simulink model "PolarCinematica2015"  (R2015a)
settings: Solver=ode45  SolverMode=SingleTasking  StartTime=0.0  StopTime=Tfinal  RelTol=1e-3
values from neighbouring files (symbols this model uses):
  Tem = 0.001    [circular.m]
undefined symbols (not defined in the file or in its folder): Diferencia, mgd_Polar, mgi_Polar
libraries: simulink x1
settings Model: CovMetricSettings=dwe  CovHtmlReporting=off  covSaveCumulativeToWorkspaceVar=off  CovSaveSingleToWorkspaceVar=off  CovExternalEMLEnable=on  Creator=Shadow  LastModifiedBy=Shadow
settings DataIOCC: LimitDataPoints=off  SaveFormat=Dataset  ReturnWorkspaceOutputs=on
settings DebuggingCC: SFUnexpectedBacktrackingDiag=error  SFNoUnconditionalDefaultTransitionDiag=error
settings HardwareCC: ProdBitPerPointer=64  ProdLargestAtomicFloat=Float  ProdIntDivRoundTo=Zero  ProdEndianess=LittleEndian  ProdHWDeviceType=Specified
settings ModelReferenceCC: PropagateSignalLabelsOutOfModel=on
settings SFSimCC: SimUseLocalCustomCode=on
settings RTWCC: RTWUseLocalCustomCode=on
settings GRTTargetCC: TargetLangStandard=C99 (ISO)

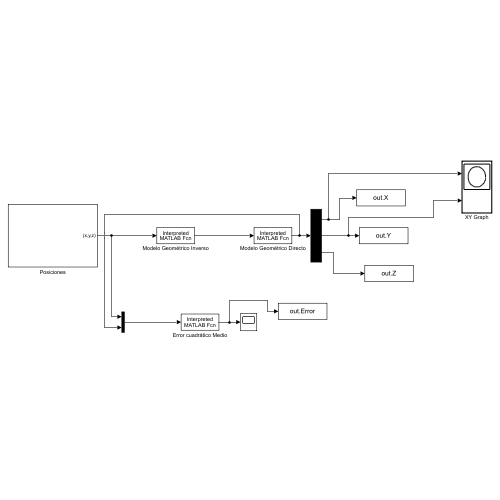
[thumbnail: Simulink's stored preview of the top-level diagram]
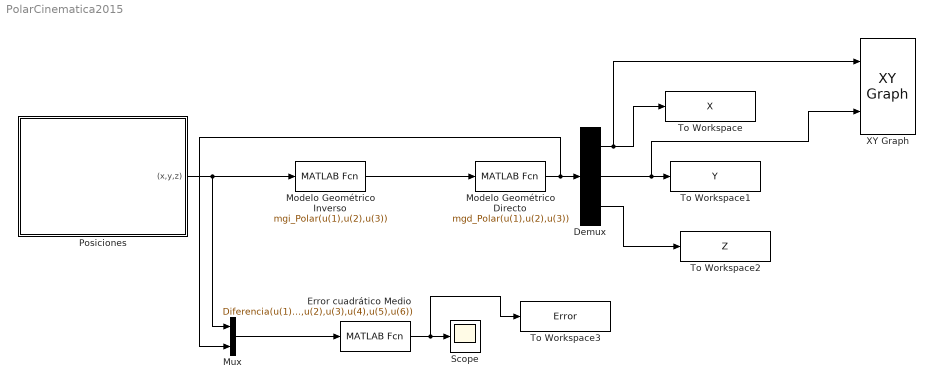
== system PolarCinematica2015 ==
  Demux : Demux  Outputs=3
  Error cuadrático Medio : MATLABFcn  MATLABFcn=Diferencia(u(1),u(2),u(3),u(4),u(5),u(6))  OutputDimensions=1
  Modelo Geométrico Directo : MATLABFcn  MATLABFcn=mgd_Polar(u(1),u(2),u(3))  OutputDimensions=3
  Modelo Geométrico Inverso : MATLABFcn  MATLABFcn=mgi_Polar(u(1),u(2),u(3))  OutputDimensions=3
  Mux : Mux  Inputs=2
  Posiciones : Subsystem
  Scope : Scope
      settings: TimeRange=auto  MaxDataPoints=5000  SaveToWorkspace=off  SaveName=ScopeData  YMin=-0.00000000000000000  YMax=0.0000000000000003  SampleTime=-1
  To Workspace : ToWorkspace  VariableName=X
  To Workspace1 : ToWorkspace  VariableName=Y
  To Workspace2 : ToWorkspace  VariableName=Z
  To Workspace3 : ToWorkspace  VariableName=Error
  XY Graph : simulink/Sinks/XY Graph  xmin=-1  xmax=1  ymin=-1  ymax=1  st=-1
  wires:
  Demux/2 -> XY Graph/2, To Workspace1/1
  Demux/3 -> To Workspace2/1
  Modelo Geométrico Inverso/1 -> Modelo Geométrico Directo/1
  Posiciones/1((x,y,z)) -> Mux/1, Modelo Geométrico Inverso/1
  Demux/1 -> To Workspace/1, XY Graph/1
  Mux/1 -> Error cuadrático Medio/1
  Modelo Geométrico Directo/1 -> Mux/2, Demux/1
  Error cuadrático Medio/1 -> To Workspace3/1, Scope/1

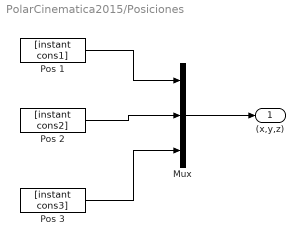
== system PolarCinematica2015/Posiciones ==
  Mux : Mux  Inputs=3
  Pos 1 : FromWorkspace  VariableName=[instant cons1]  SampleTime=Tem
  Pos 2 : FromWorkspace  VariableName=[instant cons2]  SampleTime=Tem
  Pos 3 : FromWorkspace  VariableName=[instant cons3]  SampleTime=Tem
  (x,y,z) : Outport
  wires:
  Pos 3/1 -> Mux/3
  Pos 1/1 -> Mux/1
  Pos 2/1 -> Mux/2
  Mux/1 -> (x,y,z)/1
